simulink model "EvitaParedes"  (R2023b)
settings: Solver=FixedStepAuto  StartTime=0.0  StopTime=inf  RelTol=1e-3
libraries: simulink x2
settings Model: ExtModeTrigDuration=2  Creator=Usuario_UMA  LastModifiedBy=pablo
settings SolverCC: AlgebraicLoopSolver=TrustRegion
settings OptimizationCC: EnhancedBackFolding=on  PassReuseOutputArgsAs=Individual arguments  ZeroExternalMemoryAtStartup=off  ZeroInternalMemoryAtStartup=off  MaxStackSize=64  OptimizeBlockOrder=speed  DifferentSizesBufferReuse=on  OptimizationCustomize=off  EfficientTunableParamExpr=on
settings DebuggingCC: ParameterTunabilityLossMsg=error  UnconnectedInputMsg=warning  UnconnectedOutputMsg=warning  UnconnectedLineMsg=warning
settings HardwareCC: ProdBitPerInt=16  ProdBitPerPointer=16  ProdBitPerSizeT=16  ProdBitPerPtrDiffT=16  ProdLargestAtomicFloat=None  ProdWordSize=8  ProdHWDeviceType=Atmel->AVR  UseEmbeddedCoderFeatures=off  UseSimulinkCoderFeatures=off
settings ModelReferenceCC: EnableRefExpFcnMdlSchedulingChecks=on
settings SFSimCC: MATLABDynamicMemAlloc=off
settings RTWCC: Description=Embedded Coder  SystemTargetFile=ert.tlc  HardwareBoard=Arduino Mega 2560  TemplateMakefile=ert_default_tmf  Toolchain=Arduino AVR  DLArmComputeVersion=19.05
settings CodeAppCC: ForceParamTrailComments=on  IgnoreCustomStorageClasses=off  OperatorAnnotations=on  SimulinkDataObjDesc=on  SFDataObjDesc=on  MangleLength=10  InsertBlockDesc=on
settings ERTTargetCC: SupportContinuousTime=on  SupportNonInlinedSFcns=on  SupportVariableSizeSignals=on  ExtModeTransport=3  ExtModeStaticAlloc=on  ExtModeAutomaticAllocSize=off  ExtModeStaticAllocSize=2048  ExtModeMexFile=ext_xcp  ExtModeIntrfLevel=Level2 - Open

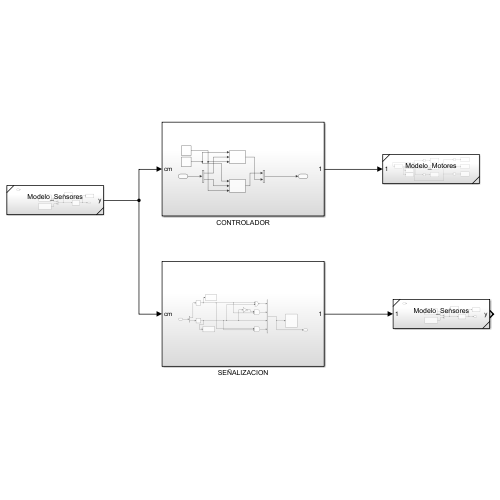
[thumbnail: Simulink's stored preview of the top-level diagram]
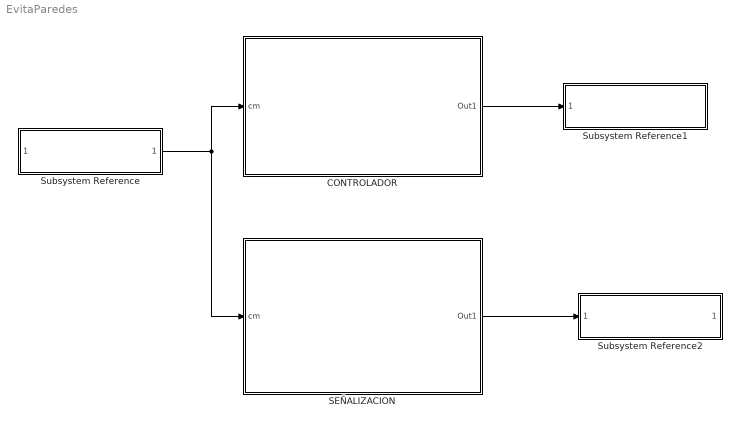
== system EvitaParedes ==
  CONTROLADOR : Subsystem
  SEÑALIZACION : Subsystem
  Subsystem Reference : Subsystem  ReferencedSubsystem=Modelo_Sensores
  Subsystem Reference1 : Subsystem  ReferencedSubsystem=Modelo_Motores
  Subsystem Reference2 : Subsystem  ReferencedSubsystem=Modelo_Sensores
  wires:
  CONTROLADOR/1(Out1) -> Subsystem Reference1/1
  Subsystem Reference/1 -> CONTROLADOR/1(cm), SEÑALIZACION/1(cm)
  SEÑALIZACION/1(Out1) -> Subsystem Reference2/1

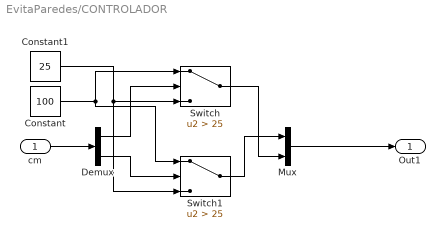
== system EvitaParedes/CONTROLADOR ==
  cm : Inport
  Constant : Constant  Value=100
  Constant1 : Constant  Value=25
  Demux : Demux  Outputs=2
  Mux : Mux  Inputs=2
  Switch : Switch  Criteria=u2 > Threshold  Threshold=25  OutDataTypeStr=int16  SaturateOnIntegerOverflow=off  InputSameDT=off
  Switch1 : Switch  Criteria=u2 > Threshold  Threshold=25  OutDataTypeStr=int16  SaturateOnIntegerOverflow=off  InputSameDT=off
  Out1 : Outport
  wires:
  cm/1 -> Demux/1
  Mux/1 -> Out1/1
  Demux/1 -> Switch/2
  Switch/1 -> Mux/2
  Demux/2 -> Switch1/2
  Switch1/1 -> Mux/1
  Constant/1 -> Switch1/1, Switch/1
  Constant1/1 -> Switch1/3, Switch/3

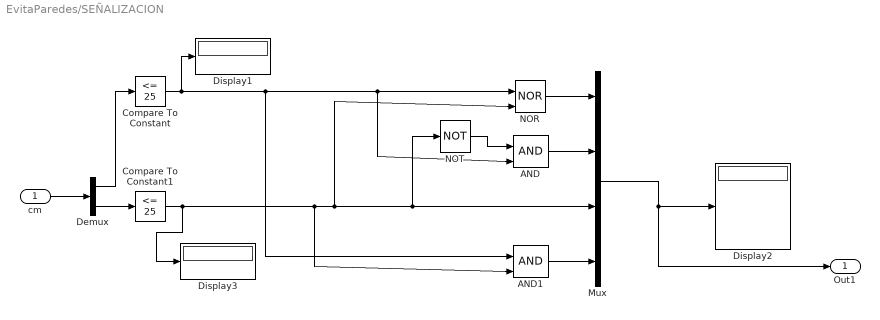
== system EvitaParedes/SEÑALIZACION ==
  cm : Inport
  AND : Logic  IconShape=distinctive  AllPortsSameDT=off  OutDataTypeStr=boolean
  AND1 : Logic  IconShape=distinctive  AllPortsSameDT=off  OutDataTypeStr=boolean
  Compare To Constant : simulink/Logic and Bit Operations/Compare To Constant  relop=<=  const=25  OutDataTypeStr=boolean
  Compare To Constant1 : simulink/Logic and Bit Operations/Compare To Constant  relop=<=  const=25  OutDataTypeStr=boolean
  Demux : Demux  Outputs=2
  Display1 : Display
  Display2 : Display
  Display3 : Display
  Mux : Mux
  NOR : Logic  Operator=NOR  IconShape=distinctive  AllPortsSameDT=off  OutDataTypeStr=boolean
  NOT : Logic  Operator=NOT  IconShape=distinctive  AllPortsSameDT=off  OutDataTypeStr=boolean
  Out1 : Outport
  wires:
  cm/1 -> Demux/1
  Demux/2 -> Compare To Constant1/1
  Demux/1 -> Compare To Constant/1
  Mux/1 -> Out1/1, Display2/1
  Compare To Constant1/1 -> Display3/1, AND1/2, NOR/2, NOT/1, Mux/3
  NOR/1 -> Mux/1
  AND/1 -> Mux/2
  AND1/1 -> Mux/4
  Compare To Constant/1 -> Display1/1, AND1/1, AND/2, NOR/1
  NOT/1 -> AND/1
